simulink model "Motorized_Pendulum_Fdbck_Lin"  (R2020b)
settings: Solver=VariableStepAuto  StartTime=0.0  StopTime=tsim  MaxStep=1e-4  MinStep=1e-6  RelTol=1e-9
undefined symbols (not defined in the file): g_n, Jm, Jp, KcRa, Km, L_n, M_n, N_n, x0
libraries: simulink_extras x3, simulink x1
settings Model: Creator=domin  LastModifiedBy=domin
settings SolverCC: ZeroCrossAlgorithm=Adaptive
settings DebuggingCC: IgnoredZcDiagnostic=none

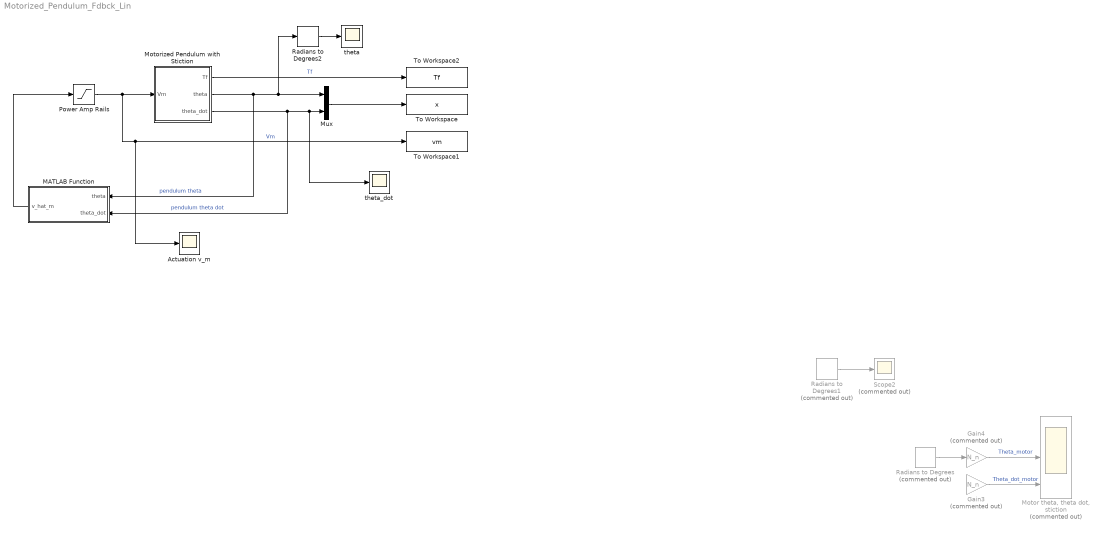
== system Motorized_Pendulum_Fdbck_Lin ==
  Actuation v_m : Scope
  Gain3 : Gain  Commented=on  Gain=N_n
  Gain4 : Gain  Commented=on  Gain=N_n
  MATLAB Function : MATLAB Function  TreatAsAtomicUnit=on
  "Motor theta, theta dot, stiction" : Scope  Commented=on  NumInputPorts=3
  Motorized Pendulum with Stiction : Subsystem
  Mux : Mux  Inputs=2
  Power Amp Rails : Saturate  UpperLimit=15  LowerLimit=-15
  Radians to Degrees : simulink_extras/Transformations/Radians to Degrees  Commented=on
  Radians to Degrees1 : simulink_extras/Transformations/Radians to Degrees  Commented=on
  Radians to Degrees2 : simulink_extras/Transformations/Radians to Degrees
  Scope2 : Scope  Commented=on
  To Workspace : ToWorkspace  VariableName=x  SampleTime=-1
  To Workspace1 : ToWorkspace  VariableName=vm  SampleTime=-1
  To Workspace2 : ToWorkspace  VariableName=Tf  SampleTime=-1
  theta : Scope
  theta_dot : Scope
  wires:
  Mux/1 -> To Workspace/1
  Power Amp Rails/1 -> Actuation v_m/1, To Workspace1/1, Motorized Pendulum with Stiction/1(Vm)  "Vm"
  Motorized Pendulum with Stiction/3(theta_dot) -> MATLAB Function/2(theta_dot), theta_dot/1, Mux/2  "pendulum theta dot"
  Motorized Pendulum with Stiction/2(theta) -> MATLAB Function/1(theta), Radians to Degrees2/1, Mux/1  "pendulum theta"
  Radians to Degrees1/1 -> Scope2/1
  Gain4/1 -> "Motor theta, theta dot, stiction"/2  "Theta_motor"
  Radians to Degrees/1 -> Gain4/1
  Gain3/1 -> "Motor theta, theta dot, stiction"/3  "Theta_dot_motor"
  Motorized Pendulum with Stiction/1(Tf) -> To Workspace2/1  "Tf"
  MATLAB Function/1(v_hat_m) -> Power Amp Rails/1
  Radians to Degrees2/1 -> theta/1

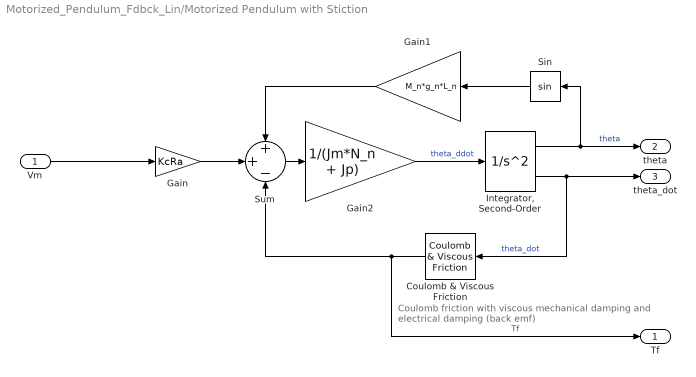
== system Motorized_Pendulum_Fdbck_Lin/Motorized Pendulum with Stiction ==
  note: Coulomb friction with viscous mechanical damping
      | and electrical damping (back emf)
  Vm : Inport
  Coulomb & Viscous Friction : simulink/Discontinuities/Coulomb & Viscous Friction  offset=T_ba_n  gain=N_n*KcRa/Km
  Gain : Gain  Gain=KcRa
  Gain1 : Gain  Gain=M_n*g_n*L_n
  Gain2 : Gain  Gain=1/(Jm*N_n + Jp)
  "Integrator, Second-Order" : SecondOrderIntegrator  ICX=x0(1)  ICDXDT=x0(2)  ZeroCross=off
  Sin : Trigonometry
  Sum : Sum  Inputs=++-
  Tf : Outport
  theta : Outport  Port=2
  theta_dot : Outport  Port=3
  wires:
  Gain2/1 -> "Integrator, Second-Order"/1  "theta_ddot"
  Sin/1 -> Gain1/1
  "Integrator, Second-Order"/2 -> theta_dot/1, Coulomb & Viscous Friction/1  "theta_dot"
  Coulomb & Viscous Friction/1 -> Tf/1, Sum/3  "Tf"
  "Integrator, Second-Order"/1 -> Sin/1, theta/1  "theta"
  Gain1/1 -> Sum/1
  Sum/1 -> Gain2/1
  Vm/1 -> Gain/1
  Gain/1 -> Sum/2

== matlab function Motorized_Pendulum_Fdbck_Lin/MATLAB Function ==
  data: theta input; theta_dot input; v_hat_m output; lambda_n parameter
function v_hat_m = fcn(theta, theta_dot, lambda_n)


v_hat_m = 0.3401*theta_dot - 1.0684*sign(theta_dot) - 0.6600*sin(theta)...
    - 0.1144*lambda_n*theta_dot;
